simulink subsystem "bounding_controller_spine"  (R2024a)
settings: Solver=VariableStepAuto  StartTime=0.0  StopTime=10.0  RelTol=1e-3
undefined symbols (not defined in the file or in its folder): Femur, Motor, Piston, Spine, Tibia
settings Model: Creator=Mechatronics  LastModifiedBy=Mechatronics

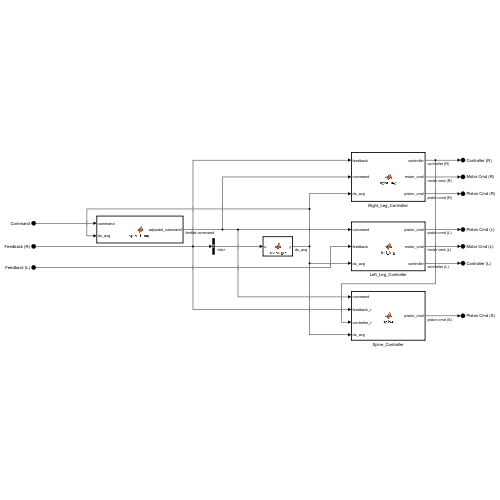
[thumbnail: Simulink's stored preview of the top-level diagram]
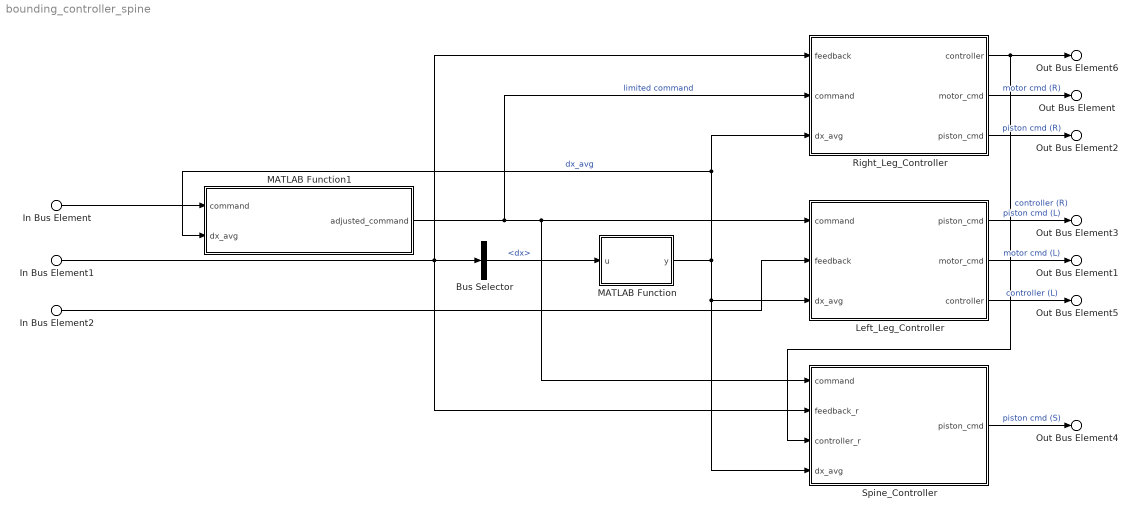
== system bounding_controller_spine ==
  In Bus Element : Inport  PortName=Command
  In Bus Element1 : Inport  Port=2  PortName=Feedback (R)
  In Bus Element2 : Inport  Port=3  PortName=Feedback (L)
  Bus Selector : BusSelector  OutputSignals=Body.dx
  Left_Leg_Controller : MATLAB Function  TreatAsAtomicUnit=on  SystemSampleTime=0.001
  MATLAB Function : MATLAB Function  TreatAsAtomicUnit=on
  MATLAB Function1 : MATLAB Function  TreatAsAtomicUnit=on
  Right_Leg_Controller : MATLAB Function  TreatAsAtomicUnit=on  SystemSampleTime=0.001
  Spine_Controller : MATLAB Function  TreatAsAtomicUnit=on  SystemSampleTime=0.001
  Out Bus Element : Outport  PortName=Motor Cmd (R)
  Out Bus Element1 : Outport  Port=2  PortName=Motor Cmd (L)
  Out Bus Element2 : Outport  Port=3  PortName=Piston Cmd (R)
  Out Bus Element3 : Outport  Port=4  PortName=Piston Cmd (L)
  Out Bus Element4 : Outport  Port=5  PortName=Piston Cmd (S)
  Out Bus Element5 : Outport  Port=6  PortName=Controller (L)
  Out Bus Element6 : Outport  Port=7  PortName=Controller (R)
  wires:
  MATLAB Function/1(y) -> Left_Leg_Controller/3(dx_avg), Spine_Controller/4(dx_avg), MATLAB Function1/2(dx_avg), Right_Leg_Controller/3(dx_avg)  "dx_avg"
  Right_Leg_Controller/1(controller) -> Spine_Controller/3(controller_r), Out Bus Element6/1  "controller (R)"
  In Bus Element1/1 -> Right_Leg_Controller/1(feedback), Bus Selector/1, Spine_Controller/2(feedback_r)
  In Bus Element2/1 -> Left_Leg_Controller/2(feedback)
  Right_Leg_Controller/2(motor_cmd) -> Out Bus Element/1  "motor cmd (R)"
  Left_Leg_Controller/2(motor_cmd) -> Out Bus Element1/1  "motor cmd (L)"
  Right_Leg_Controller/3(piston_cmd) -> Out Bus Element2/1  "piston cmd (R)"
  Left_Leg_Controller/1(piston_cmd) -> Out Bus Element3/1  "piston cmd (L)"
  Spine_Controller/1(piston_cmd) -> Out Bus Element4/1  "piston cmd (S)"
  Left_Leg_Controller/3(controller) -> Out Bus Element5/1  "controller (L)"
  Bus Selector/1 -> MATLAB Function/1(u)  "<dx>"
  In Bus Element/1 -> MATLAB Function1/1(command)
  MATLAB Function1/1(adjusted_command) -> Right_Leg_Controller/2(command), Spine_Controller/1(command), Left_Leg_Controller/1(command)  "limited command"

== matlab function bounding_controller_spine/Right_Leg_Controller ==
  data: controller output Bus: Controller; feedback input; motor_cmd output Bus: MotorCmd; piston_cmd output Bus: PistonCmd; command input Bus: Command; Femur parameter; Tibia parameter; Piston parameter; Motor parameter; Spine parameter; dx_avg input
function [controller, motor_cmd, piston_cmd] = right_leg(feedback, command, Femur, Tibia, Piston, Motor, Spine,dx_avg)

% initialisation
hip.y = 0; hip.dy = 0; hip.y_min = 0; hip.y_max = 0;
foot.y = 0; foot.height = 0; foot.contact = false; foot.radius = 20e-3;

motor = feedback.Motor;
pistonLeg = feedback.PistonLeg;
body = feedback.Body;
pistonSpine = feedback.PistonSpine;

body.dx = dx_avg;

mass_leg = Femur.Right.mass + Tibia.mass + Piston.Body.mass + Piston.Rod.mass + Motor.Cover.mass;
mass_body_right = Spine.RightBody.mass + Spine.PistonRod.mass + 0.5*Spine.LeftBody.mass + 0.5*Spine.PistonBody.mass;
mass_pointR = mass_leg + mass_body_right;
Fe_static = 324;

% kinematics
[r,dr,phi,dphi] = virtural_leg_f(pistonLeg.v, body.dr, motor.w, pistonLeg.p, body.r, motor.q);
[~, ~ ,hip.y, hip.dy] = hip_pos_f(pistonSpine.v, body.dr, body.dx, body.dy, pistonSpine.p, body.r, body.x, body.y);
[~,foot.y] = foot_pos_f(pistonLeg.p, pistonSpine.p, body.r, motor.q, body.x, body.y);

% constants
command.height = min(command.height + 0.03*body.dx,0.39);
contact_threshold = 5e-3; % m relies on ground being flat
contact_acceleration_threshold = -100; %-100; % m/s^2
retract_duration = 17;% + 1*body.dx; % 17ms
hip.amplitude = 0.04;
hip.y_min = min(command.height - 0.5*hip.amplitude,0.35);%+ 0.006*body.dx);
hip.y_max = command.height + 0.5*hip.amplitude;

kdx = 0.1;

persistent state
persistent retract_timer
persistent ground_offset
persistent Ts

if isempty(state)
    state = States.Rest;
end
if isempty(retract_timer)
    retract_timer = 0;
end
if isempty(ground_offset)
    ground_offset = 0;
end
if isempty(Ts)
    Ts = 0;
end

% contact detection
foot.height = foot.y + ground_offset;
if foot.height > contact_threshold
    foot.contact = false;
else
    foot.contact = true;
end
 
% state transitions
switch(state)
    case States.Rest
        if command.start
            state = States.Stance;
            ground_offset = -foot.y;
        end
    case States.Flight
        if ((hip.y + ground_offset) < ((mass_pointR*hip.dy*hip.dy)/(2*(Fe_static - 9.81*mass_pointR)) + hip.y_min)) && (hip.dy < 0)
            state = States.Loading;
        elseif (hip.y_min < 0.17) && (command.stop)
            state = States.Rest;
        end
    case States.Loading
        if pistonLeg.a < contact_acceleration_threshold
            Ts = 0;
            state = States.Stance;
        end
    case States.Stance
        if hip.dy > 0
            if (hip.y + ground_offset) > ((hip.dy*hip.dy)/(-2*9.81) + hip.y_max)
                retract_timer = 0;
                ground_offset = -foot.y; % update ground offset
                state = States.Unloading;
            end
        end
    case States.Unloading
        % if ~foot.contact
        %     state = States.Flight;
        % end
        if retract_duration < retract_timer
            state = States.Flight;
        end
end
 
 
% control piston
switch(state)
    case {States.Loading, States.Stance}
        piston_cmd.ue = 1;
        piston_cmd.ur = 0;
    case States.Unloading
        piston_cmd.ue = 0;
        if retract_timer < retract_duration
            piston_cmd.ur = 1;
        else
            piston_cmd.ur = 0;
        end
        retract_timer = retract_timer + 1;
    case States.Flight
        if ((foot.height-0.1)<=0)
            piston_cmd.ue = 0;
            piston_cmd.ur = 1;
        else
            piston_cmd.ue = 0;
            piston_cmd.ur = 0;
        end
    otherwise
        piston_cmd.ue = 0;
        piston_cmd.ur = 0;
end

% stance timer
switch(state)
    case {States.Stance, States.Unloading}
        Ts = Ts + 0.001;
end

% control motor
foot_offset = 0;
switch(state)
    case States.Loading
        foot_offset = (Ts*body.dx)/(2) + kdx*(body.dx -  command.speed);
        foot_offset = max(min(foot_offset,0.04),-0.1);
        phi_d = -pi/2 + asin(foot_offset/r);
        dphi_d = (dr*cos(phi) + command.speed)/(r*sin(phi));
        Kp = 10; % 80
        Kd = 4; % 2
    case {States.Stance, States.Unloading}
        phi_d = -pi/2;
        dphi_d = (dr*cos(phi) + command.speed)/(r*sin(phi));
        Kp = 0;
        Kd = 4;
    case {States.Flight}
        foot_offset = (Ts*body.dx)/(2) + kdx*(body.dx -  command.speed);
        foot_offset = max(min(foot_offset,0.04),-1)+0.03*body.dx;
        phi_d = -pi/2 + asin(min(foot_offset,r)/r);
        dphi_d = 0;
        Kp = 100; % 80
        Kd = 4; % 2
    otherwise
        phi_d = -pi/2;
        dphi_d = 0;
        Kp = 50;
        Kd = 4;
end

[theta_m_des, dtheta_m_des] = phi_tracking_f(pistonLeg.v, dphi_d, body.dr, pistonLeg.p, phi_d, body.r);
% bound motor angle to not break pneumatics
theta_m_des = max(-pi, theta_m_des);

motor_cmd.q = theta_m_des;
motor_cmd.w = dtheta_m_des;
motor_cmd.Kp = Kp;
motor_cmd.Kd = Kd;
motor_cmd.tff = 0;

controller.state = state; controller.Ts = Ts;
 
end

== matlab function bounding_controller_spine/Left_Leg_Controller ==
  data: command input Bus: Command; piston_cmd output Bus: PistonCmd; motor_cmd output Bus: MotorCmd; feedback input; controller output Bus: Controller; Femur parameter; Tibia parameter; Piston parameter; Motor parameter; Spine parameter; dx_avg input
function [piston_cmd, motor_cmd, controller] = left_leg(command, feedback, Femur, Tibia, Piston, Motor, Spine,dx_avg)

% initialisation
hip.y = 0; hip.dy = 0; hip.y_min = 0; hip.y_max = 0;
foot.y = 0; foot.height = 0; foot.contact = false; foot.radius = 20e-3;

mass_leg = Femur.Left.mass + Tibia.mass + Piston.Body.mass + Piston.Rod.mass + Motor.Cover.mass;
% mass_body_left = 0.5*(Spine.LeftBack.mass + Spine.LeftFront.mass) + 0.5*Spine.Body.mass + 2*Spine.EndStop.mass + Spine.Mounting.mass + Spine.Spacer.mass + 2*Spine.PTFE.mass;
mass_body_left = 0.5*Spine.LeftBody.mass + 0.5*Spine.PistonBody.mass;
mass_pointL = mass_leg + mass_body_left;
% mass_pointL = 2.137;
% mass_pointL = 2.5;
Fe_static = 324;

motor = feedback.Motor;
piston = feedback.PistonLeg;
body = feedback.Body;

body.dx = dx_avg;

% Fe_static = 324*cos(motor.q + 0.5);

% % constants
command.height = min(command.height + 0.03*body.dx,0.39);
contact_threshold = 5e-3; % m foot radius
contact_acceleration_threshold = -100; % m/s^2
retract_duration = 17;% + 1*body.dx; % 17ms
hip.amplitude = 0.025;
hip.y_min = min(command.height - 0.5*hip.amplitude,0.35);% + 0.006*body.dx);
hip.y_max = command.height + 0.5*hip.amplitude;

kdx = 0.1;

% kinematics
[r,dr,phi,~] = virtural_leg_b(piston.v, body.dr, motor.w, piston.p, body.r, motor.q);
[~, ~ ,hip.y, hip.dy] = hip_pos_b(body.dr, body.dx, body.dy, body.r, body.x, body.y);
[~,foot.y] = foot_pos_b(piston.p, body.r, motor.q, body.x, body.y);

persistent state
persistent retract_timer
persistent ground_offset
persistent Ts
if isempty(state)
    state = States.Rest;
end
if isempty(retract_timer)
    retract_timer = 0;
end
if isempty(ground_offset)
    ground_offset = 0;
end
if isempty(Ts)
    Ts = 0;
end

% contact detection
foot.height = foot.y + ground_offset;
if foot.height > contact_threshold
    foot.contact = false;
else
    foot.contact = true;
end

% state transitions
switch(state)
    case States.Rest
        if (body.r > 0.1) && (command.start) % wait until right leg has pushed off a bit
            state = States.Stance;
            ground_offset = -foot.y;
        end
    case States.Flight
        if ((hip.y + ground_offset) < ((mass_pointL*hip.dy*hip.dy)/(2*(Fe_static - 9.81*mass_pointL)) + hip.y_min)) && (hip.dy < 0)
            state = States.Loading;
        elseif (hip.y_min < 0.17) && (command.stop)
            state = States.Rest;
        end
    case States.Loading
        if piston.a < contact_acceleration_threshold
            Ts = 0;
            state = States.Stance;
        end
    case States.Stance
        if hip.dy > 0
            if (hip.y + ground_offset) > ((hip.dy*hip.dy)/(-2*9.81) + hip.y_max)
                retract_timer = 0;
                ground_offset = -foot.y; % update ground offset
                state = States.Unloading;
            end
        end
    case States.Unloading
        % if ~foot.contact
        %     state = States.Flight;
        % end
        if retract_duration < retract_timer
            state = States.Flight;
        end
end


% control piston
switch(state)
    case {States.Loading, States.Stance}
        piston_cmd.ue = 1;
        piston_cmd.ur = 0;
    case States.Unloading
        piston_cmd.ue = 0;
        if retract_timer < retract_duration
            piston_cmd.ur = 1;
        else
            piston_cmd.ur = 0;
        end
        retract_timer = retract_timer + 1;
    case States.Flight
        if ((foot.height-0.05)<=0)
            piston_cmd.ue = 0;
            piston_cmd.ur = 1;
        else
            piston_cmd.ue = 0;
            piston_cmd.ur = 0;
        end
    otherwise
        piston_cmd.ue = 0;
        piston_cmd.ur = 0;
end

% stance timer
switch(state)
    case {States.Stance, States.Unloading}
        Ts = Ts + 0.001;
end

% control motor
foot_offset = 0;
switch(state)
    case States.Loading
        foot_offset = (Ts*body.dx)/(2) + kdx*(body.dx -  command.speed);
        foot_offset = max(min(foot_offset,0.04),-1);
        phi_d = -pi/2 + asin(foot_offset/r);
        dphi_d = (dr*cos(phi) + command.speed)/(r*sin(phi));
        Kp = 20; % 80
        Kd = 4; % 2
    case {States.Stance, States.Unloading}
        phi_d = -pi/2;
        dphi_d = (dr*cos(phi) + command.speed)/(r*sin(phi));
        Kp = 0;
        Kd = 4;
    case {States.Flight}
        foot_offset = (Ts*body.dx)/(2) + kdx*(body.dx -  command.speed);
        foot_offset = max(min(foot_offset,0.04),-1)+0.03*body.dx;
        phi_d = -pi/2 + asin(min(foot_offset,r)/r);
        dphi_d = 0;
        Kp = 100; % 80
        Kd = 4; % 2
    otherwise
        phi_d = -pi/2;
        dphi_d = 0;
        Kp = 50;
        Kd = 4;
end
 
[theta_m_des,dtheta_m_des] = phi_tracking_b(piston.v, dphi_d, body.dr, piston.p, phi_d, body.r);
% bound motor angle to not break pneumatics
theta_m_des =  min(theta_m_des, 0);

motor_cmd.q = theta_m_des;
motor_cmd.w = dtheta_m_des;
motor_cmd.Kp = Kp;
motor_cmd.Kd = Kd;
motor_cmd.tff = 0;

controller.state = state; controller.Ts = Ts;
 
end

== matlab function bounding_controller_spine/Spine_Controller ==
  data: command input Bus: Command; piston_cmd output Bus: PistonCmd; feedback_r input; controller_r input; dx_avg input
function piston_cmd = spine(command, feedback_r,controller_r,dx_avg) %

% initialisation
piston_s = feedback_r.PistonSpine;
state = controller_r.state;
Ts = controller_r.Ts;

offset_max = 0.04; %max forward offset of foot before spine starts actuating initially was 0.26

persistent flight_time %time foot is in flight. Currently static but should be changed to be dynamic
persistent spine_stop; % trigger if spine is over limit. Needs to be built into states. 1 is actuate, 2 is rest, 0 is retract

if(isempty(spine_stop))
    spine_stop = 0;
end

if isempty(flight_time)
    flight_time = 0.08;
end

% get xf of front leg
kdx = 0.1;
foot_offset = (Ts*dx_avg)/(2) + kdx*(dx_avg -  command.speed);

% for now 0 = extend; 1 = stop extending; 2 = retracted

% state transitions
switch(spine_stop)
    case 0
        if (foot_offset>offset_max&&(state == States.Unloading || state == States.Flight))
            spine_stop = 1;
        end
    case 1
        if piston_s.v >= (foot_offset-offset_max-piston_s.p)/(flight_time)
            spine_stop = 2;
        end
    case 2
        if (state == States.Loading || state == States.Stance || state == States.Rest)
            spine_stop = 0;
        end
end

switch(spine_stop)
    case 0
        piston_cmd.ue = 0;
        piston_cmd.ur = 1;
    case 1
        piston_cmd.ue = 1;
        piston_cmd.ur = 0;
    case 2
        piston_cmd.ue = 0;
        piston_cmd.ur = 0;
    otherwise
        piston_cmd.ue = 0;
        piston_cmd.ur = 0;
end

end

== matlab function bounding_controller_spine/MATLAB Function ==
  data: u input; y output
function y = average(u)

changing = 0.005;
persistent avg

if isempty(avg)
    avg = 0;
end

avg = avg*(1-changing) + u*changing;

y = avg;

== matlab function bounding_controller_spine/MATLAB Function1 ==
  data: command input Bus: Command; adjusted_command output Bus: Command; dx_avg input
function adjusted_command =speed_cap(command,dx_avg)

persistent speed_out latch

if isempty(speed_out)
    speed_out = 0;
end

if isempty(latch)
    latch = 0;
end

if latch == 0
    if (command.speed<2.55)
        speed_out = command.speed;
    else
        latch = 1;
    end
else
    if dx_avg > 3.1
        speed_out = speed_out - 0.0001;
    elseif command.speed < 2.4
        latch = 0;
    end
end

command.speed = speed_out;

adjusted_command = command;
